simulink model "Simulator_Case_7"  (R2024a)
settings: Solver=VariableStepAuto  StartTime=0.0  StopTime=1000  RelTol=1e-3
values from neighbouring files (symbols this model uses):
  Declination_Sigean = 2.116*(pi/180)    (= 0.0369311669722)    [Parametrization_Simulation_Case_7.m]
  Position_Initial_X = Waypoints_X(1)    [Parametrization_Simulation_Case_7.m]
  Position_Initial_Y = Waypoints_Y(1)    [Parametrization_Simulation_Case_7.m]
  Time_Guidance_Sampling = 20    [Parametrization_Simulation_Case_7.m]
  Time_Period_Sampling = 0.1    [Parametrization_Simulation_Case_7.m]
undefined symbols (not defined in the file or in its folder): Area_Lateral_Projected_Wind, Damping_Factor_Waves, Density_Air, Gain_Derivative, Gain_Filter, Gain_Proportional, Inertia_Moment, Length_Ship, Pulsation_Wave, Rudder_Angle_Maximal, Rudder_Angle_Minimal, Rudder_Rate_Maximal, Rudder_Rate_Minimal, Static_Gain_Nomoto, Structure_Wind_Coefficient, Time_Constant_Total, Velocity_Ship_Mean, Wave_Transfer_Function_Discrete, Waypoints, Yaw_Control_Hydrodynamics_Derivative
libraries: simulink_extras x6, cstblocks x2, sensorgpslib x1, sensorinslib x1
(part 2 of 2)

== matlab function Simulator_Case_7/Navigation_And_Wave_Estimator/Sensors_Fusion_And_Filtering/Kinematics_Propagator_GPS ==
  settings: updateMethod=DISCRETE
  data: Velocity_Current input; Heading_Angle_Current_Mes input; Position_X_Ship_Init input; Position_Y_Ship_Init input; Time_Simulation_Current input; Position_X_Ship_Compass_Next output; Position_Y_Ship_Compass_Next output; Acceleration_X_Ship_Next output; Acceleration_Y_Ship_Next output; Velocity_X_Ship_Next_Local output; Velocity_Y_Ship_Next_Local output; Time_Sampling input
function [Position_X_Ship_Compass_Next,...
          Position_Y_Ship_Compass_Next,...
          Acceleration_X_Ship_Next,...
          Acceleration_Y_Ship_Next,...
          Velocity_X_Ship_Next_Local,...
          Velocity_Y_Ship_Next_Local] = Kinematics_Propagation(Velocity_Current,...
                                                               Heading_Angle_Current_Mes,...
                                                               Position_X_Ship_Init,...
                                                               Position_Y_Ship_Init,...
                                                               Time_Simulation_Current,...
                                                               Time_Sampling)

% Persistents definition:
persistent Position_X_Ship_Compass_Prev
persistent Position_Y_Ship_Compass_Prev
persistent Heading_Previous
persistent Velocity_X_Ship_Local_Previous
persistent Velocity_Y_Ship_Local_Previous

% Heading previous storage:
if isempty(Heading_Previous)
    Heading_Previous = Heading_Angle_Current_Mes;
    Heading_Current = Heading_Previous;
else
    Heading_Current = Heading_Angle_Current_Mes;
end

% Calculate the local position increment but use both convention (unit and compass):
% Compass:
Position_X_Ship_Current_Increment_Compass = Time_Sampling*Velocity_Current*sin(Heading_Previous);
Position_Y_Ship_Current_Increment_Compass = Time_Sampling*Velocity_Current*cos(Heading_Previous);

% The simple velocity discrete increment:
Velocity_X_Ship_Local = Velocity_Current*sin(Heading_Angle_Current_Mes);
Velocity_Y_Ship_Local = Velocity_Current*cos(Heading_Angle_Current_Mes);

if isempty(Velocity_X_Ship_Local_Previous)
    Velocity_X_Ship_Local_Previous = Velocity_Current*sin(Heading_Angle_Current_Mes);
    Acceleration_X_Ship_Next = 0;
else
    Acceleration_X_Ship_Next = (Velocity_X_Ship_Local - Velocity_X_Ship_Local_Previous)/Time_Sampling;
    Velocity_X_Ship_Local_Previous = Velocity_X_Ship_Local;
end
if isempty(Velocity_Y_Ship_Local_Previous)
    Velocity_Y_Ship_Local_Previous = Velocity_Current*cos(Heading_Angle_Current_Mes);
    Acceleration_Y_Ship_Next = 0;
else
    Acceleration_Y_Ship_Next = (Velocity_Y_Ship_Local - Velocity_Y_Ship_Local_Previous)/Time_Sampling;
    Velocity_Y_Ship_Local_Previous = Velocity_Y_Ship_Local;
end


% Compass position persistent filling:
if isempty(Position_X_Ship_Compass_Prev)
    Position_X_Ship_Compass_Prev = Position_X_Ship_Init + Position_X_Ship_Current_Increment_Compass;
else
    Position_X_Ship_Compass_Prev = Position_X_Ship_Compass_Prev + Position_X_Ship_Current_Increment_Compass;
end
if isempty(Position_Y_Ship_Compass_Prev)
    Position_Y_Ship_Compass_Prev = Position_Y_Ship_Init + Position_Y_Ship_Current_Increment_Compass;
else
    Position_Y_Ship_Compass_Prev = Position_Y_Ship_Compass_Prev + Position_Y_Ship_Current_Increment_Compass;
end

% Then update the outputs:
% Compass:
Position_X_Ship_Compass_Next = Position_X_Ship_Compass_Prev;
Position_Y_Ship_Compass_Next = Position_Y_Ship_Compass_Prev;

% Store the heading:
Heading_Estimated_Next = Heading_Current;
Heading_Previous = Heading_Estimated_Next;

% Velocity:
Velocity_X_Ship_Next_Local = Velocity_X_Ship_Local;
Velocity_Y_Ship_Next_Local = Velocity_Y_Ship_Local;

end

== matlab function Simulator_Case_7/Navigation_And_Wave_Estimator/Wave_Estimation_Kalman_Filter/Wave_Heading_Estimation ==
  data: Heading_Total_Observed_Current input; Rudder_Angle_Commanded_Current input; Wave_Pulsation_Estimated input; Damping_Wave_Estimated input; Time_Current input; Time_Constant_Ship input; Gain_Ship input; Time_Sampling input; Noise_For_Heading_wave input; Heading_Rate_Wave_Estimated_Current output; Heading_Wave_Estimated_Current output; Heading_Low_Frequency_Estimated_Current output; Heading_Rate_Estimated_Current output; Bias_Estimated_Current output; Covariance_Aposteriori_Estimate output; Torque_Wind_Estimated_Input input; Inertia_Ship_Vertical input; Wave_Pulsation_Identified input
function [Heading_Rate_Wave_Estimated_Current,...
          Heading_Wave_Estimated_Current,...
          Heading_Low_Frequency_Estimated_Current,...
          Heading_Rate_Estimated_Current,...
          Bias_Estimated_Current,...
          Covariance_Aposteriori_Estimate]= Kalman_Filter_Wave_Estimation(Heading_Total_Observed_Current,...
                                                                          Rudder_Angle_Commanded_Current,...
                                                                          Wave_Pulsation_Estimated,...
                                                                          Damping_Wave_Estimated,...
                                                                          Time_Current,...
                                                                          Time_Constant_Ship,...
                                                                          Gain_Ship,...
                                                                          Time_Sampling,...
                                                                          Noise_For_Heading_wave,...
                                                                          Torque_Wind_Estimated_Input,...
                                                                          Inertia_Ship_Vertical,...
                                                                          Wave_Pulsation_Identified)

% Online Wave Observer Kalman algorithm for better wave high frequency
% filtering:
[Heading_Rate_Wave_Estimated_Current,...
 Heading_Wave_Estimated_Current,...
 Heading_Low_Frequency_Estimated_Current,...
 Heading_Rate_Estimated_Current,...
 Bias_Estimated_Current,...
 Covariance_Aposteriori_Estimate] = Kalman_Observer_Wave_Estimation(Heading_Total_Observed_Current,...
                                                                    Rudder_Angle_Commanded_Current,...
                                                                    Wave_Pulsation_Estimated,...
                                                                    Damping_Wave_Estimated,...
                                                                    Time_Current,...
                                                                    Time_Constant_Ship,...
                                                                    Gain_Ship,...
                                                                    Time_Sampling,...
                                                                    Noise_For_Heading_wave,...
                                                                    Torque_Wind_Estimated_Input,...
                                                                    Inertia_Ship_Vertical,...
                                                                    Wave_Pulsation_Identified);

end
